simulink model "bacteriaPopulationDemo"  (R2017b)
settings: Solver=FixedStepDiscrete  StartTime=0.0  StopTime=10.0  FixedStep=1  RelTol=1e-3
model workspace (MAT data in the model file):
  ContractValidatorBlocksMap = containers.Map
  ContractValidatorBlocksMap.serialization.keys = {'bacteriaPopulation/bacteriaPopulationSpec/validator', 'bacteriaPopulation/contract/validator'}
  ContractValidatorBlocksMap.serialization.values{1}.block = 'bacteriaPopulation/bacteriaPopulationSpec/validator'
  ContractValidatorBlocksMap.serialization.values{1}.assumePorts = 1
  ContractValidatorBlocksMap.serialization.values{1}.guaranteePorts = 4
  ContractValidatorBlocksMap.serialization.values{1}.modeBlocksPorts = 3
  ContractValidatorBlocksMap.serialization.values{1}.portHandles.Inport = [341.00769043 342.008300781 343.008056641 344.009521484 345.009155273 346.008911133 347.007568359 348.01574707]
  ContractValidatorBlocksMap.serialization.values{1}.portHandles.Outport = 349.009643555
  ContractValidatorBlocksMap.serialization.values{1}.portHandles.Enable = []
  ContractValidatorBlocksMap.serialization.values{1}.portHandles.Trigger = []
  ContractValidatorBlocksMap.serialization.values{1}.portHandles.State = []
  ContractValidatorBlocksMap.serialization.values{1}.portHandles.LConn = []
  ContractValidatorBlocksMap.serialization.values{1}.portHandles.RConn = []
  ContractValidatorBlocksMap.serialization.values{1}.portHandles.Ifaction = []
  ContractValidatorBlocksMap.serialization.values{1}.portHandles.Reset = []
  ContractValidatorBlocksMap.serialization.values{1}.portConnectivity(1).Type = '1'
  ContractValidatorBlocksMap.serialization.values{1}.portConnectivity(1).Position = [360 -280]
  ContractValidatorBlocksMap.serialization.values{1}.portConnectivity(1).SrcBlock = 53.0080566406
  ContractValidatorBlocksMap.serialization.values{1}.portConnectivity(1).SrcPort = 0
  ContractValidatorBlocksMap.serialization.values{1}.portConnectivity(1).DstBlock = []
  ContractValidatorBlocksMap.serialization.values{1}.portConnectivity(1).DstPort = []
  ContractValidatorBlocksMap.serialization.values{1}.portConnectivity(2).Type = '2'
  ContractValidatorBlocksMap.serialization.values{1}.portConnectivity(2).Position = [360 -170]
  ContractValidatorBlocksMap.serialization.values{1}.portConnectivity(2).SrcBlock = 113.006225586
  ContractValidatorBlocksMap.serialization.values{1}.portConnectivity(2).SrcPort = 0
  ContractValidatorBlocksMap.serialization.values{1}.portConnectivity(2).DstBlock = []
  ContractValidatorBlocksMap.serialization.values{1}.portConnectivity(2).DstPort = []
  ContractValidatorBlocksMap.serialization.values{1}.portConnectivity(3).Type = '3'
  ContractValidatorBlocksMap.serialization.values{1}.portConnectivity(3).Position = [360 -60]
  ContractValidatorBlocksMap.serialization.values{1}.portConnectivity(3).SrcBlock = 119.006713867
  ContractValidatorBlocksMap.serialization.values{1}.portConnectivity(3).SrcPort = 0
  ContractValidatorBlocksMap.serialization.values{1}.portConnectivity(3).DstBlock = []
  ContractValidatorBlocksMap.serialization.values{1}.portConnectivity(3).DstPort = []
  ContractValidatorBlocksMap.serialization.values{1}.portConnectivity(4).Type = '4'
  ContractValidatorBlocksMap.serialization.values{1}.portConnectivity(4).Position = [360 50]
  ContractValidatorBlocksMap.serialization.values{1}.portConnectivity(4).SrcBlock = 131.005859375
  ContractValidatorBlocksMap.serialization.values{1}.portConnectivity(4).SrcPort = 0
  ContractValidatorBlocksMap.serialization.values{1}.portConnectivity(4).DstBlock = []
  ContractValidatorBlocksMap.serialization.values{1}.portConnectivity(4).DstPort = []
  ContractValidatorBlocksMap.serialization.values{1}.portConnectivity(5).Type = '5'
  ContractValidatorBlocksMap.serialization.values{1}.portConnectivity(5).Position = [360 160]
  ContractValidatorBlocksMap.serialization.values{1}.portConnectivity(5).SrcBlock = 180.006347656
  ContractValidatorBlocksMap.serialization.values{1}.portConnectivity(5).SrcPort = 0
  ContractValidatorBlocksMap.serialization.values{1}.portConnectivity(5).DstBlock = []
  ContractValidatorBlocksMap.serialization.values{1}.portConnectivity(5).DstPort = []
  ContractValidatorBlocksMap.serialization.values{1}.portConnectivity(6).Type = '6'
  ContractValidatorBlocksMap.serialization.values{1}.portConnectivity(6).Position = [360 270]
  ContractValidatorBlocksMap.serialization.values{1}.portConnectivity(6).SrcBlock = 229.007568359
  ContractValidatorBlocksMap.serialization.values{1}.portConnectivity(6).SrcPort = 0
  ContractValidatorBlocksMap.serialization.values{1}.portConnectivity(6).DstBlock = []
  ContractValidatorBlocksMap.serialization.values{1}.portConnectivity(6).DstPort = []
  ContractValidatorBlocksMap.serialization.values{1}.portConnectivity(7).Type = '7'
  ContractValidatorBlocksMap.serialization.values{1}.portConnectivity(7).Position = [360 380]
  ContractValidatorBlocksMap.serialization.values{1}.portConnectivity(7).SrcBlock = 59.0084228516
  ContractValidatorBlocksMap.serialization.values{1}.portConnectivity(7).SrcPort = 0
  ContractValidatorBlocksMap.serialization.values{1}.portConnectivity(7).DstBlock = []
  ContractValidatorBlocksMap.serialization.values{1}.portConnectivity(7).DstPort = []
  ContractValidatorBlocksMap.serialization.values{1}.portConnectivity(8).Type = '8'
  ContractValidatorBlocksMap.serialization.values{1}.portConnectivity(8).Position = [360 490]
  ContractValidatorBlocksMap.serialization.values{1}.portConnectivity(8).SrcBlock = 270.005249023
  ContractValidatorBlocksMap.serialization.values{1}.portConnectivity(8).SrcPort = 0
  ContractValidatorBlocksMap.serialization.values{1}.portConnectivity(8).DstBlock = []
  ContractValidatorBlocksMap.serialization.values{1}.portConnectivity(8).DstPort = []
  ContractValidatorBlocksMap.serialization.values{1}.portConnectivity(9).Type = '1'
  ContractValidatorBlocksMap.serialization.values{1}.portConnectivity(9).Position = [500 105]
  ContractValidatorBlocksMap.serialization.values{1}.portConnectivity(9).SrcBlock = []
  ContractValidatorBlocksMap.serialization.values{1}.portConnectivity(9).SrcPort = []
  ContractValidatorBlocksMap.serialization.values{1}.portConnectivity(9).DstBlock = [282.008911133 52.0072021484]
  ContractValidatorBlocksMap.serialization.values{1}.portConnectivity(9).DstPort = [0 0]
  ContractValidatorBlocksMap.serialization.values{2}.block = 'bacteriaPopulation/contract/validator'
  ContractValidatorBlocksMap.serialization.values{2}.assumePorts = 1
  ContractValidatorBlocksMap.serialization.values{2}.guaranteePorts = 3
  ContractValidatorBlocksMap.serialization.values{2}.modeBlocksPorts = 2
  ContractValidatorBlocksMap.serialization.values{2}.portHandles.Inport = [450.00012207 448.00012207 449.00012207 454.00012207 451.00012207 456.00012207]
  ContractValidatorBlocksMap.serialization.values{2}.portHandles.Outport = 445.00012207
  ContractValidatorBlocksMap.serialization.values{2}.portHandles.Enable = []
  ContractValidatorBlocksMap.serialization.values{2}.portHandles.Trigger = []
  ContractValidatorBlocksMap.serialization.values{2}.portHandles.State = []
  ContractValidatorBlocksMap.serialization.values{2}.portHandles.LConn = []
  ContractValidatorBlocksMap.serialization.values{2}.portHandles.RConn = []
  ContractValidatorBlocksMap.serialization.values{2}.portHandles.Ifaction = []
  ContractValidatorBlocksMap.serialization.values{2}.portHandles.Reset = []
  ContractValidatorBlocksMap.serialization.values{2}.portConnectivity(1).Type = '1'
  ContractValidatorBlocksMap.serialization.values{2}.portConnectivity(1).Position = [365 -135]
  ContractValidatorBlocksMap.serialization.values{2}.portConnectivity(1).SrcBlock = 458.00012207
  ContractValidatorBlocksMap.serialization.values{2}.portConnectivity(1).SrcPort = 0
  ContractValidatorBlocksMap.serialization.values{2}.portConnectivity(1).DstBlock = []
  ContractValidatorBlocksMap.serialization.values{2}.portConnectivity(1).DstPort = []
  ContractValidatorBlocksMap.serialization.values{2}.portConnectivity(2).Type = '2'
  ContractValidatorBlocksMap.serialization.values{2}.portConnectivity(2).Position = [365 -50]
  ContractValidatorBlocksMap.serialization.values{2}.portConnectivity(2).SrcBlock = 462.00012207
  ContractValidatorBlocksMap.serialization.values{2}.portConnectivity(2).SrcPort = 0
  ContractValidatorBlocksMap.serialization.values{2}.portConnectivity(2).DstBlock = []
  ContractValidatorBlocksMap.serialization.values{2}.portConnectivity(2).DstPort = []
  ContractValidatorBlocksMap.serialization.values{2}.portConnectivity(3).Type = '3'
  ContractValidatorBlocksMap.serialization.values{2}.portConnectivity(3).Position = [365 35]
  ContractValidatorBlocksMap.serialization.values{2}.portConnectivity(3).SrcBlock = 465.000366211
  ContractValidatorBlocksMap.serialization.values{2}.portConnectivity(3).SrcPort = 0
  ContractValidatorBlocksMap.serialization.values{2}.portConnectivity(3).DstBlock = []
  ContractValidatorBlocksMap.serialization.values{2}.portConnectivity(3).DstPort = []
  ContractValidatorBlocksMap.serialization.values{2}.portConnectivity(4).Type = '4'
  ContractValidatorBlocksMap.serialization.values{2}.portConnectivity(4).Position = [365 120]
  ContractValidatorBlocksMap.serialization.values{2}.portConnectivity(4).SrcBlock = 478.00012207
  ContractValidatorBlocksMap.serialization.values{2}.portConnectivity(4).SrcPort = 0
  ContractValidatorBlocksMap.serialization.values{2}.portConnectivity(4).DstBlock = []
  ContractValidatorBlocksMap.serialization.values{2}.portConnectivity(4).DstPort = []
  ContractValidatorBlocksMap.serialization.values{2}.portConnectivity(5).Type = '5'
  ContractValidatorBlocksMap.serialization.values{2}.portConnectivity(5).Position = [365 205]
  ContractValidatorBlocksMap.serialization.values{2}.portConnectivity(5).SrcBlock = 503.000366211
  ContractValidatorBlocksMap.serialization.values{2}.portConnectivity(5).SrcPort = 0
  ContractValidatorBlocksMap.serialization.values{2}.portConnectivity(5).DstBlock = []
  ContractValidatorBlocksMap.serialization.values{2}.portConnectivity(5).DstPort = []
  ContractValidatorBlocksMap.serialization.values{2}.portConnectivity(6).Type = '6'
  ContractValidatorBlocksMap.serialization.values{2}.portConnectivity(6).Position = [365 290]
  ContractValidatorBlocksMap.serialization.values{2}.portConnectivity(6).SrcBlock = 526.000610352
  ContractValidatorBlocksMap.serialization.values{2}.portConnectivity(6).SrcPort = 0
  ContractValidatorBlocksMap.serialization.values{2}.portConnectivity(6).DstBlock = []
  ContractValidatorBlocksMap.serialization.values{2}.portConnectivity(6).DstPort = []
  ContractValidatorBlocksMap.serialization.values{2}.portConnectivity(7).Type = '1'
  ContractValidatorBlocksMap.serialization.values{2}.portConnectivity(7).Position = [500 80]
  ContractValidatorBlocksMap.serialization.values{2}.portConnectivity(7).SrcBlock = []
  ContractValidatorBlocksMap.serialization.values{2}.portConnectivity(7).SrcPort = []
  ContractValidatorBlocksMap.serialization.values{2}.portConnectivity(7).DstBlock = 438.00012207
  ContractValidatorBlocksMap.serialization.values{2}.portConnectivity(7).DstPort = 0
  ContractValidatorBlocksMap.serialization.uniformity = 0
  ContractValidatorBlocksMap.serialization.keyType = 'char'
  ContractValidatorBlocksMap.serialization.valueType = 'any'
libraries: simulink x2, Kind x1
settings Model: Creator=mahgoubyahia  LastModifiedBy=Mudathir
settings OptimizationCC: LifeSpan=inf
settings DebuggingCC: SFExecutionAtInitializationDiag=none
settings HardwareCC: ProdBitPerSizeT=32  ProdBitPerPtrDiffT=32  ProdWordSize=32  ProdHWDeviceType=Specified
settings CodeAppCC: StateflowObjectComments=on

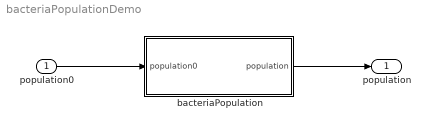
== system bacteriaPopulationDemo ==
  population0 : Inport
  bacteriaPopulation : Subsystem
  population : Outport
  wires:
  population0/1 -> bacteriaPopulation/1(population0)
  bacteriaPopulation/1(population) -> population/1

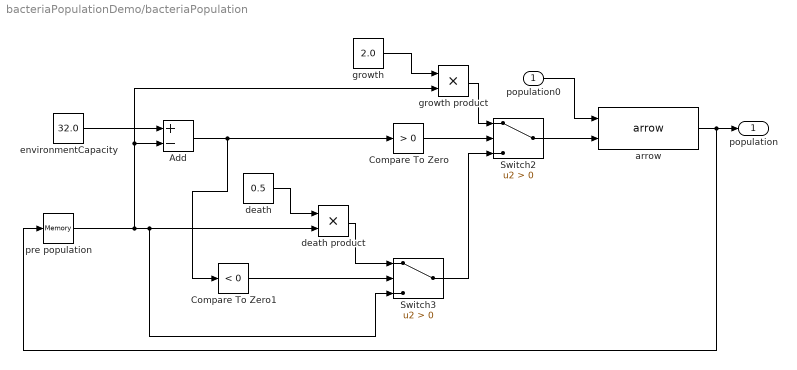
== system bacteriaPopulationDemo/bacteriaPopulation ==
  population0 : Inport
  Add : Sum  Inputs=+-
  Compare To Zero : simulink/Logic and Bit Operations/Compare To Zero  relop=>  OutDataTypeStr=boolean
  Compare To Zero1 : simulink/Logic and Bit Operations/Compare To Zero  relop=<  OutDataTypeStr=boolean
  Switch2 : Switch  Criteria=u2 > Threshold
  Switch3 : Switch  Criteria=u2 > Threshold
  arrow : Kind/arrow  LustreOperatorBlock=ArrowOperator
  death : Constant  Value=0.5  OutDataTypeStr=double
  death product : Product
  environmentCapacity : Constant  Value=32.0  OutDataTypeStr=double
  growth : Constant  Value=2.0  OutDataTypeStr=double
  growth product : Product
  pre population : Memory
  population : Outport
  wires:
  growth/1 -> growth product/1
  Add/1 -> Compare To Zero1/1, Compare To Zero/1
  growth product/1 -> Switch2/1
  Compare To Zero1/1 -> Switch3/2
  environmentCapacity/1 -> Add/1
  Compare To Zero/1 -> Switch2/2
  Switch3/1 -> Switch2/3
  Switch2/1 -> arrow/2
  pre population/1 -> Switch3/3, death product/2, Add/2, growth product/2
  population0/1 -> arrow/1
  death/1 -> death product/1
  death product/1 -> Switch3/1
  arrow/1 -> pre population/1, population/1
